simulink model "ograniczenie_pwm"  (Simulink 8.4)
settings: Solver=ode45  StartTime=0.0  StopTime=10.0  RelTol=1e-3
settings Model: Creator=Michal  LastModifiedBy=Michal
settings DataIOCC: SignalLoggingSaveFormat=Dataset
settings OptimizationCC: ExpressionDepthLimit=128
settings DebuggingCC: UnderspecifiedInitializationDetection=Simplified  MergeDetectMultiDrivingBlocksExec=error  FcnCallInpInsideContextMsg=EnableAllAsError  StateNameClashWarn=none
settings GRTTargetCC: CombineOutputUpdateFcns=on  GRTInterface=off
settings ConfigComp: Description=PLC Coder Custom Configuration Component  PLC_TargetIDE=pcworx60  PLC_GenerateReport=off

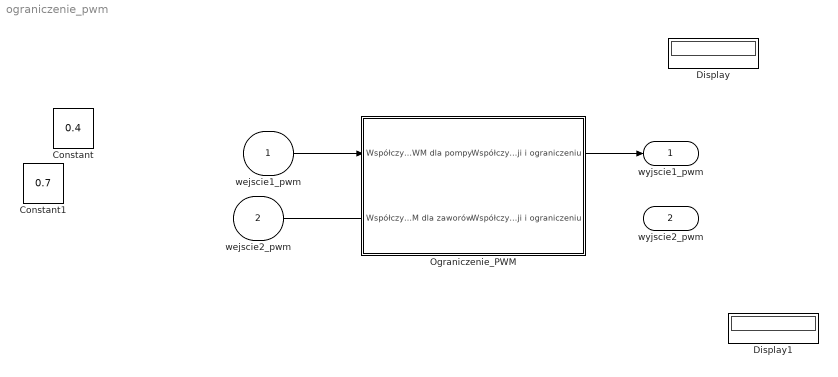
== system ograniczenie_pwm ==
  wejscie1_pwm : Inport  OutDataTypeStr=single
  wejscie2_pwm : Inport  Port=2  OutDataTypeStr=single
  Constant : Constant  Value=0.4  OutDataTypeStr=single
  Constant1 : Constant  Value=0.7  OutDataTypeStr=single
  Display : Display
  Display1 : Display
  "Ograniczenie_PWM " : Subsystem  TreatAsAtomicUnit=on
      settings: MinAlgLoopOccurrences=on
  wyjscie1_pwm : Outport  OutDataTypeStr=uint32
  wyjscie2_pwm : Outport  Port=2  OutDataTypeStr=uint32
  wires:
  "Ograniczenie_PWM "/1(Współczynnik wypełnienia sygnału PWM dla pompy  po konwersji i ograniczeniu) -> wyjscie1_pwm/1
  ? -> wyjscie2_pwm/1
  wejscie1_pwm/1 -> "Ograniczenie_PWM "/1(Współczynnik wypełnienia sygnału PWM dla pompy)
  wejscie2_pwm/1 -> ?

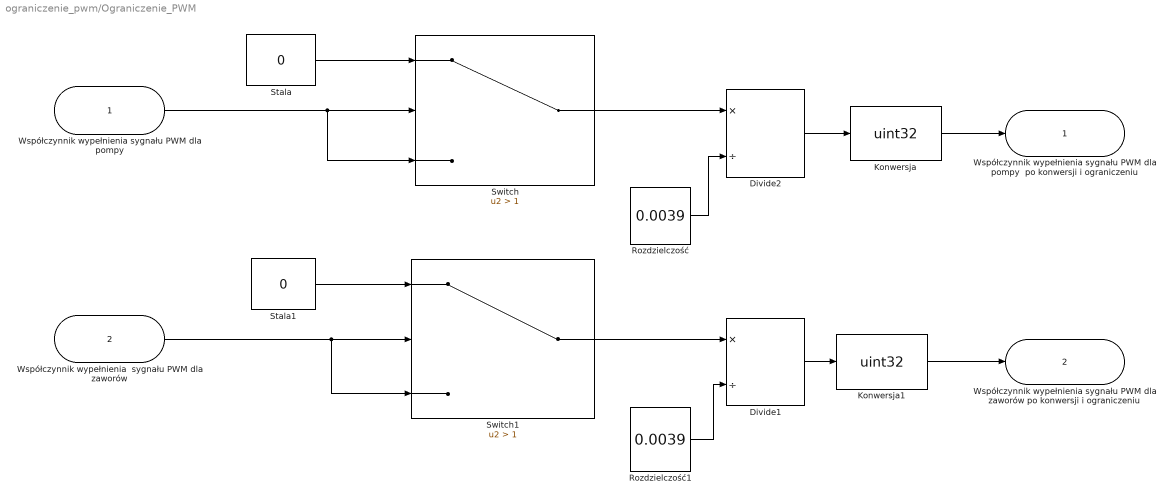
== system ograniczenie_pwm/Ograniczenie_PWM  ==
  Współczynnik wypełnienia sygnału PWM dla pompy : Inport  OutDataTypeStr=single
  "Współczynnik wypełnienia  sygnału PWM dla zaworów " : Inport  Port=2  OutDataTypeStr=single
  Divide1 : Product  Inputs=*/
  Divide2 : Product  Inputs=*/
  Konwersja : DataTypeConversion  OutDataTypeStr=uint32
  Konwersja1 : DataTypeConversion  OutDataTypeStr=uint32
  Rozdzielczość : Constant  Value=0.0039  OutDataTypeStr=single
  Rozdzielczość1 : Constant  Value=0.0039  OutDataTypeStr=single
  Stala : Constant  Value=0  OutDataTypeStr=single
  Stala1 : Constant  Value=0  OutDataTypeStr=single
  Switch : Switch  Criteria=u2 > Threshold  Threshold=1
  Switch1 : Switch  Criteria=u2 > Threshold  Threshold=1
  Współczynnik wypełnienia sygnału PWM dla pompy  po konwersji i ograniczeniu : Outport  OutDataTypeStr=uint32
  Współczynnik wypełnienia sygnału PWM dla zaworów po konwersji i ograniczeniu : Outport  Port=2  OutDataTypeStr=uint32
  wires:
  Stala1/1 -> Switch1/1
  Stala/1 -> Switch/1
  "Współczynnik wypełnienia  sygnału PWM dla zaworów "/1 -> Switch1/3, Switch1/2
  Konwersja/1 -> Współczynnik wypełnienia sygnału PWM dla pompy  po konwersji i ograniczeniu/1
  Switch/1 -> Divide2/1
  Divide2/1 -> Konwersja/1
  Rozdzielczość/1 -> Divide2/2
  Divide1/1 -> Konwersja1/1
  Rozdzielczość1/1 -> Divide1/2
  Switch1/1 -> Divide1/1
  Konwersja1/1 -> Współczynnik wypełnienia sygnału PWM dla zaworów po konwersji i ograniczeniu/1
  Współczynnik wypełnienia sygnału PWM dla pompy/1 -> Switch/3, Switch/2
